simulink model "acc_sim"  (R2022b)
settings: Solver=ode4  StartTime=0.0  StopTime=Tf  FixedStep=Tc  RelTol=1e-3
undefined symbols (not defined in the file): Kd, Ki, Kp, tau, Vx_d, Vx_i
settings Model: Creator=user  LastModifiedBy=user
settings DataIOCC: ReturnWorkspaceOutputs=off

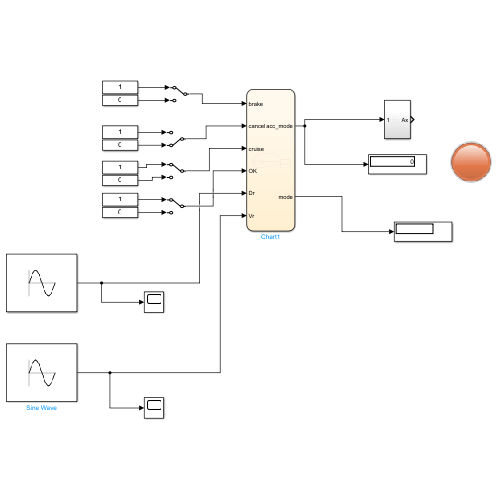
[thumbnail: Simulink's stored preview of the top-level diagram]
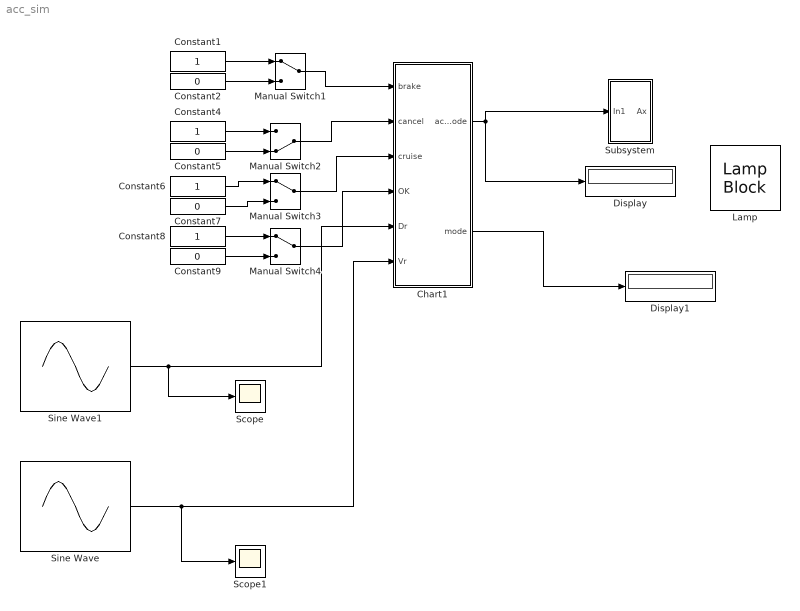
== system acc_sim ==
  Chart1 : Stateflow chart  TreatAsAtomicUnit=on
      settings: PortSchema="{\"entries\":[{\"content\":{\"sides\":[{\"content\":{\"connectorIds\":[\"In2\",\"In3\",\"In1\",\"In4\",\"In5\",\"In6\"]},\"type\":\"ConnectorPlacement.EquallySpacedRectSide\",\"uuid\":\"7a5e9d17-ec92-4b7a-8eec-ec7a76394c58\"},{\"content\":{\"connectorIds\":[\"Out1\",\"Out2\"],\"side\":\"RIGHT\"},\"type\":\"ConnectorPlacement.EquallySpacedRectSide\",\"uuid\":\"379bef9b-74df-4834-a283-668696636535\"},{\"content\":{\"connectorIds\":[],\"side\":\"TOP\"},\"type\":\"ConnectorPlacement.EquallySpacedRectSide\",\"uuid\":\"cb1e32e2-e5e4-4c3f-a6c0-cedaf2cba0f0\"}]},\"type\":\"ConnectorPlacement.EquallySpacedConnector\",\"uuid\":\"2bdc2602-a74c-4135-aa21-5d44b9f12efb\"}],\"packageUris\":[\"http://schema.mathworks.com/mf0/Connector/R2020b\"],\"version\":\"1.0\"}"
  Constant{1,4,6,8} (4 alike) : Constant
  Constant{2,5,7,9} (4 alike) : Constant  Value=0
  Display : Display
  Display1 : Display
  Lamp : LampBlock  LabelPosition=Hide
  Manual Switch1 : ManualSwitch
  Manual Switch2 : ManualSwitch  CurrentSetting=0
  Manual Switch3 : ManualSwitch
  Manual Switch4 : ManualSwitch
  Scope : Scope
  Scope1 : Scope
  Sine Wave : Sin  SampleTime=0
  Sine Wave1 : Sin  Amplitude=50  Bias=250  Frequency=0.1  SampleTime=0
  Subsystem : Subsystem
  wires:
  Chart1/1(acc_mode) -> Subsystem/1(In1), Display/1
  Constant1/1 -> Manual Switch1/1
  Constant2/1 -> Manual Switch1/2
  Constant4/1 -> Manual Switch2/1
  Constant5/1 -> Manual Switch2/2
  Constant6/1 -> Manual Switch3/1
  Constant7/1 -> Manual Switch3/2
  Constant8/1 -> Manual Switch4/1
  Constant9/1 -> Manual Switch4/2
  Manual Switch1/1 -> Chart1/2(brake)
  Manual Switch2/1 -> Chart1/3(cancel)
  Manual Switch3/1 -> Chart1/1(cruise)
  Manual Switch4/1 -> Chart1/4(OK)
  Chart1/2(mode) -> Display1/1
  Sine Wave/1 -> Scope1/1, Chart1/6(Vr)
  Sine Wave1/1 -> Scope/1, Chart1/5(Dr)

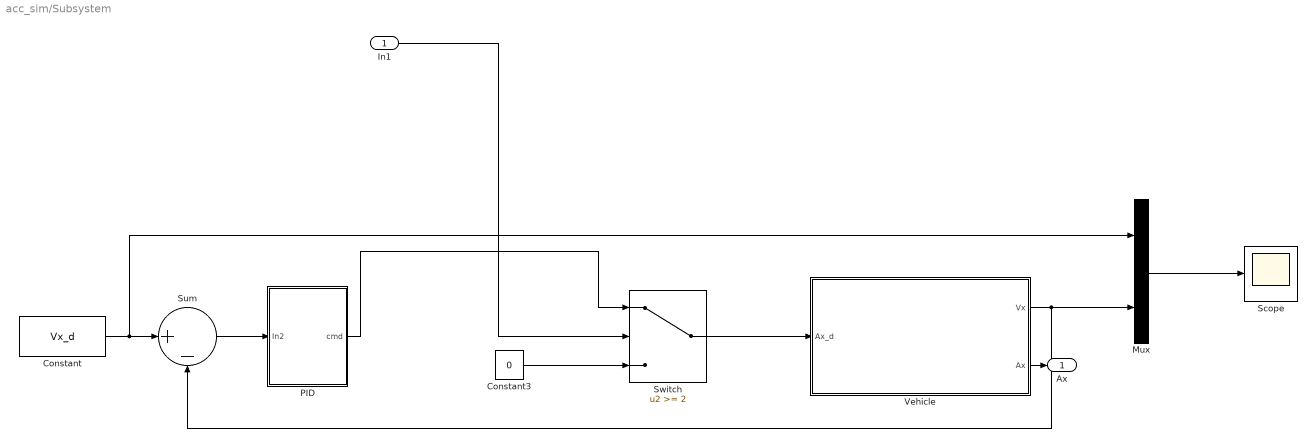
== system acc_sim/Subsystem ==
  In1 : Inport
  Constant : Constant  Value=Vx_d
  Constant3 : Constant  Value=0
  Mux : Mux  Inputs=2
  PID : Subsystem
  Scope : Scope
  Sum : Sum  Inputs=|+-
  Switch : Switch  Threshold=2  SaturateOnIntegerOverflow=off  InputSameDT=off
  Vehicle : Subsystem
  Ax : Outport
  wires:
  Mux/1 -> Scope/1
  Switch/1 -> Vehicle/1(Ax_d)
  Vehicle/2(Ax) -> Ax/1
  Constant/1 -> Mux/1, Sum/1
  Vehicle/1(Vx) -> Sum/2, Mux/2
  Sum/1 -> PID/1(In2)
  PID/1(cmd) -> Switch/1
  Constant3/1 -> Switch/3
  In1/1 -> Switch/2

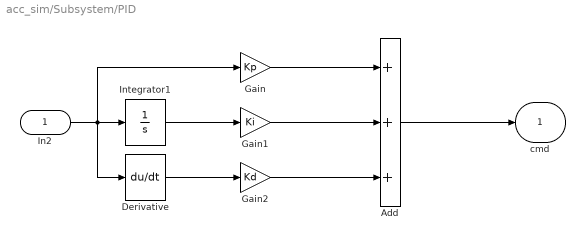
== system acc_sim/Subsystem/PID ==
  In2 : Inport
  Add : Sum  Inputs=+++
  Derivative : Derivative
  Gain : Gain  Gain=Kp
  Gain1 : Gain  Gain=Ki
  Gain2 : Gain  Gain=Kd
  Integrator1 : Integrator
  cmd : Outport
  wires:
  Add/1 -> cmd/1
  In2/1 -> Gain/1, Derivative/1, Integrator1/1
  Derivative/1 -> Gain2/1
  Gain2/1 -> Add/3
  Integrator1/1 -> Gain1/1
  Gain/1 -> Add/1
  Gain1/1 -> Add/2

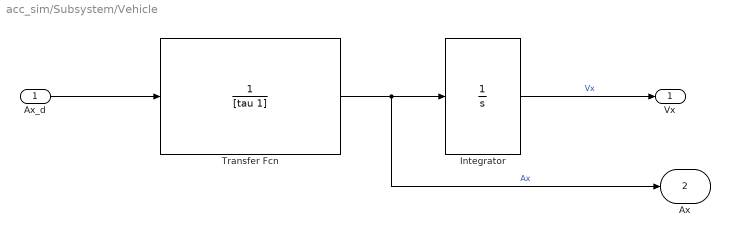
== system acc_sim/Subsystem/Vehicle ==
  Ax_d : Inport
  Integrator : Integrator  InitialCondition=Vx_i
  Transfer Fcn : TransferFcn  Denominator=[tau 1]
  Vx : Outport
  Ax : Outport  Port=2
  wires:
  Transfer Fcn/1 -> Ax/1, Integrator/1  "Ax"
  Ax_d/1 -> Transfer Fcn/1
  Integrator/1 -> Vx/1  "Vx"

== stateflow chart acc_sim/Chart1 ==
  state ACC_active
    acc_mode=2;
    state CC [parallel]
      mode = 1;
      settings: executionOrder=1
    state CTG [parallel]
      mode = 2;
      settings: executionOrder=2
    (default) -> CC
    CTG -> CC : [Vr >= 0 | Dr >= 250]
    CC -> CTG : [Vr < 0 & Dr < 250]
  state ACC_off
    acc_mode=0;
  state ACC_standby
    acc_mode=1;
  ACC_active -> ACC_off [order 2] : [cruise == 0]
  (default) -> ACC_off
  ACC_off -> ACC_standby : [cruise == 1 & brake ~= 1]
  ACC_standby -> ACC_active [order 2] : [OK == 1 & brake ~= 1]
  ACC_active -> ACC_standby [order 1] : [cancel ==1 ]
  ACC_standby -> ACC_off [order 1] : [cruise == 0]
  ACC_active -> ACC_off [order 3] : [brake == 1]
  ACC_standby -> ACC_off [order 3] : [brake == 1]
  data: cruise input; brake input; cancel input; OK input; acc_mode output; mode output; Dr input; Vr input
